simulink model "simulink_RR_adaptive"  (R2024a)
settings: Solver=FixedStepAuto  StartTime=0.0  StopTime=T_max  FixedStep=ST  RelTol=1e-3
values from neighbouring files (symbols this model uses):
  A_m = eye(2)    [init_RR.m]
  alfa = 1    [init_RR.m]
  B_m = eye(2)    [init_RR.m]
  c_11_init = ones(n_q1*n_q2,1)/(n_q1*n_q2)    [init_RR.m]
  c_12_init = ones(n_q1*n_q2,1)/(n_q1*n_q2)    [init_RR.m]
  c_21_init = ones(n_q1*n_q2,1)/(n_q1*n_q2)    [init_RR.m]
  c_22_init = ones(n_q1*n_q2,1)/(n_q1*n_q2)    [init_RR.m]
  delta_q1 = 2*1.1*q_limit/(n_q1-1)    [basis_figure.m]    (also in init_RR.m = 0.345575191895)
  delta_q2 = 2*1.1*q_limit/(n_q2-1)    [basis_figure.m]    (also in init_RR.m = 0.345575191895)
  gamma = 100    [init_RR.m]
  k_m = 1    [init_RR.m]
  k_r = 10    [init_RR.m]
  ksi_m_init = [(l1+l2)/sqrt(2); 0]    [init_RR.m]
  l1 = 4    [init_RR.m]
  l2 = 3    [init_RR.m]
  M = 1000    [init_RR.m]
  mu = 1    [init_RR.m]
  n_q1 = 3    [basis_figure.m]    (also in init_RR.m = 21)
  n_q2 = 3    [basis_figure.m]    (also in init_RR.m = 21)
  omega_r_1 = 5*2*pi/T_ref    (= 0.261799387799)    [init_RR.m]
  omega_r_2 = 7*2*pi/T_ref    (= 0.366519142919)    [init_RR.m]
  q_init = [-pi/4; +pi/4]    [init_RR.m]
  shift1 = ceil(n_q1/2)    [basis_figure.m]    (also in init_RR.m)
  shift2 = ceil(n_q2/2)    [basis_figure.m]    (also in init_RR.m)
  T_max = 300    [init_RR.m]
  u_sat = 5    [init_RR.m]
  VAR_inv = inv(VAR)    [basis_figure.m]    (also in init_RR.m)
settings Model: Creator=gabri  LastModifiedBy=gabri

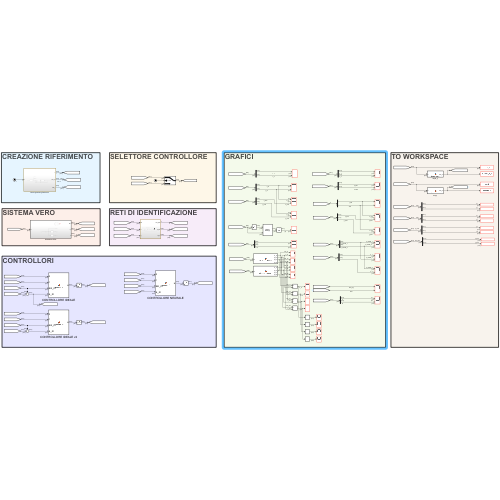
[thumbnail: Simulink's stored preview of the top-level diagram]
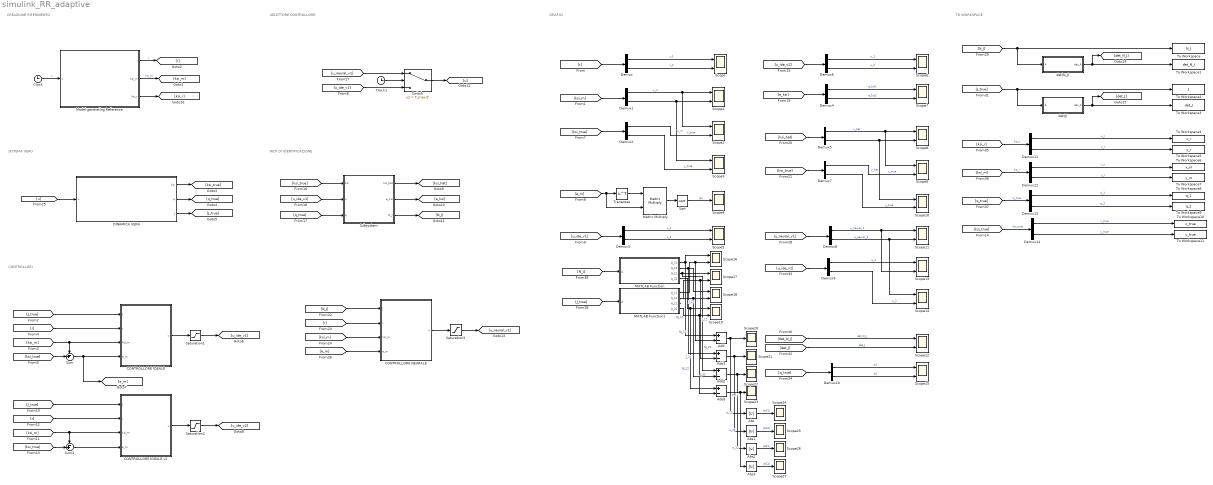
== system simulink_RR_adaptive ==
  note: TO WORKSPACE
  note: CREAZIONE RIFERIMENTO
  note: GRAFICI
  note: SISTEMA VERO
  note: CONTROLLORI
  note: SELETTORE CONTROLLORE
  note: RETI DI IDENTIFICAZIONE
  Abs{,1..3} (4 alike) : Abs  SaturateOnIntegerOverflow=off
  Add{,1..3} (4 alike) : Sum  Inputs=+-
  CONTROLLORE IDEALE : MATLAB Function  TreatAsAtomicUnit=on
  CONTROLLORE IDEALE v2 : MATLAB Function  TreatAsAtomicUnit=on
  CONTROLLORE NEURALE : MATLAB Function  TreatAsAtomicUnit=on
  Clock : Clock
  Clock1 : Clock
  DINAMICA VERA : Subsystem
  Demux{,1..14} (15 alike) : Demux  Outputs=2
  MATLAB Function : MATLAB Function  TreatAsAtomicUnit=on
  MATLAB Function1 : MATLAB Function  TreatAsAtomicUnit=on
  Matrix Multiply : Product  Multiplication=Matrix(*)
  Model generating Reference : Subsystem
  Saturation1 : Saturate  UpperLimit=u_sat  LowerLimit=-u_sat
  Saturation2 : Saturate  UpperLimit=u_sat  LowerLimit=-u_sat
  Saturation3 : Saturate  UpperLimit=u_sat  LowerLimit=-u_sat
  Scope{,1..3,5..19} (19 alike) : Scope  NumInputPorts=2
  Scope{4,20..27} (9 alike) : Scope
  Sqrt : Sqrt
  Subsystem : Subsystem
  Sum : Sum  Inputs=-+|
  Sum1 : Sum  Inputs=-+|
  Switch : Switch  Criteria=u2 > Threshold  Threshold=T_max/2  SaturateOnIntegerOverflow=off  InputSameDT=off
  To Workspace : ToWorkspace  VariableName=N_J  SaveFormat=Timeseries  SampleTime=-1
  To Workspace1 : ToWorkspace  VariableName=det_N_J  SaveFormat=Timeseries  SampleTime=-1
  To Workspace10 : ToWorkspace  VariableName=x_true  SaveFormat=Timeseries  SampleTime=-1
  To Workspace11 : ToWorkspace  VariableName=y_true  SaveFormat=Timeseries  SampleTime=-1
  To Workspace2 : ToWorkspace  VariableName=J  SaveFormat=Timeseries  SampleTime=-1
  To Workspace3 : ToWorkspace  VariableName=det_J  SaveFormat=Timeseries  SampleTime=-1
  To Workspace4 : ToWorkspace  VariableName=x_r  SaveFormat=Timeseries  SampleTime=-1
  To Workspace5 : ToWorkspace  VariableName=y_r  SaveFormat=Timeseries  SampleTime=-1
  To Workspace6 : ToWorkspace  VariableName=x_m  SaveFormat=Timeseries  SampleTime=-1
  To Workspace7 : ToWorkspace  VariableName=y_m  SaveFormat=Timeseries  SampleTime=-1
  To Workspace8 : ToWorkspace  VariableName=q_1  SaveFormat=Timeseries  SampleTime=-1
  To Workspace9 : ToWorkspace  VariableName=q_2  SaveFormat=Timeseries  SampleTime=-1
  Transpose : Math  Operator=transpose
  det(J) : MATLAB Function  TreatAsAtomicUnit=on
  det(N_J) : MATLAB Function  TreatAsAtomicUnit=on
  wires:
  Model generating Reference/2(ksi_m) -> [ksi_m]  "ksi_m"
  Model generating Reference/1(r) -> [r]  "r"
  Clock/1 -> Model generating Reference/1(t)  "t"
  Demux/1 -> Scope/1  "r_1"
  Demux/2 -> Scope/2  "r_2"
  [r] -> Demux/1
  [ksi_m] -> Demux1/1
  Demux1/2 -> Scope3/1, Scope1/2  "y_m"
  Demux1/1 -> Scope2/1, Scope1/1  "x_m"
  [u] -> DINAMICA VERA/1(u)
  DINAMICA VERA/1(ksi) -> [ksi_true]
  DINAMICA VERA/2(q) -> [q_true]
  DINAMICA VERA/3(J) -> [J_true]
  [J_true] -> CONTROLLORE IDEALE/1(J)
  [ksi_m] -> Sum/1, CONTROLLORE IDEALE/3(ksi_m)
  [r] -> CONTROLLORE IDEALE/2(r)
  [ksi_true] -> Sum/2
  Sum/1 -> [e_m], CONTROLLORE IDEALE/4(e_m)
  [u_ide_v1] -> Switch/3
  Switch/1 -> [u]
  [u_neural_v1] -> Switch/1
  [ksi_true] -> Demux2/1
  Demux2/1 -> Scope2/2  "x_true"
  Demux2/2 -> Scope3/2  "y_true"
  [e_m] -> Matrix Multiply/2, Transpose/1
  Transpose/1 -> Matrix Multiply/1
  Matrix Multiply/1 -> Sqrt/1
  Sqrt/1 -> Scope4/1  "|e|"
  [u_ide_v1] -> Demux3/1
  Demux3/1 -> Scope5/1  "u_1"
  Demux3/2 -> Scope5/2  "u_2"
  Sum1/1 -> CONTROLLORE IDEALE v2/4(e_m)
  [ksi_true] -> Sum1/2
  [r] -> CONTROLLORE IDEALE v2/2(r)
  [ksi_m] -> CONTROLLORE IDEALE v2/3(ksi_m), Sum1/1
  [J_true] -> CONTROLLORE IDEALE v2/1(J)
  Demux6/2 -> Scope6/2  "u_2"
  Demux6/1 -> Scope6/1  "u_1"
  [u_ide_v2] -> Demux6/1
  CONTROLLORE IDEALE v2/1(u) -> Saturation2/1
  CONTROLLORE IDEALE/1(u) -> Saturation1/1
  Saturation1/1 -> [u_ide_v1]
  Saturation2/1 -> [u_ide_v2]
  [ksi_true] -> Subsystem/1(ksi)
  [u_ide_v1] -> Subsystem/2(u)
  [q_true] -> Subsystem/3(q)
  Subsystem/1(ksi_hat) -> [ksi_hat]
  Subsystem/2(e_ksi) -> [e_ksi]
  Subsystem/3(N_J) -> [N_J]
  [e_ksi] -> Demux4/1
  Demux4/1 -> Scope7/1  "e_ksi1"
  Demux4/2 -> Scope7/2  "e_ksi2"
  Demux7/2 -> Scope10/2  "y_true"
  Demux7/1 -> Scope9/2  "x_true"
  [ksi_true] -> Demux7/1
  Demux5/1 -> Scope8/1, Scope9/1  "x_hat"
  Demux5/2 -> Scope8/2, Scope10/1  "y_hat"
  [ksi_hat] -> Demux5/1
  Saturation3/1 -> [u_neural_v1]
  CONTROLLORE NEURALE/1(u) -> Saturation3/1
  [N_J] -> CONTROLLORE NEURALE/1(J)
  [r] -> CONTROLLORE NEURALE/2(r)
  [ksi_m] -> CONTROLLORE NEURALE/3(ksi_m)
  [e_m] -> CONTROLLORE NEURALE/4(e_m)
  Clock1/1 -> Switch/2
  Demux8/2 -> Scope11/2, Scope14/1  "u_neural_2"
  Demux8/1 -> Scope13/2, Scope11/1  "u_neural_1"
  [u_neural_v1] -> Demux8/1
  [N_J] -> To Workspace/1, det(N_J)/1(A)
  det(N_J)/1(det_A) -> [det_N_J], To Workspace1/1
  [det_N_J] -> Scope12/1  "det_N_J"
  det(J)/1(det_A) -> To Workspace3/1, [det_J]
  [J_true] -> det(J)/1(A), To Workspace2/1
  [det_J] -> Scope12/2  "det_J"
  Demux9/2 -> Scope14/2  "u_2"
  Demux9/1 -> Scope13/1  "u_1"
  [u_ide_v1] -> Demux9/1
  [q_true] -> Demux10/1
  Demux10/1 -> Scope15/1  "q1"
  Demux10/2 -> Scope15/2  "q2"
  Model generating Reference/3(ksi_r) -> [ksi_r]
  [ksi_r] -> Demux11/1  "ksi_r"
  Demux11/2 -> To Workspace5/1  "y_r"
  Demux11/1 -> To Workspace4/1  "x_r"
  Demux12/1 -> To Workspace6/1  "x_r"
  Demux12/2 -> To Workspace7/1  "y_r"
  [ksi_m] -> Demux12/1  "ksi_r"
  [q_true] -> Demux13/1  "q_true"
  Demux13/1 -> To Workspace8/1  "q_1"
  Demux13/2 -> To Workspace9/1  "q_2"
  Demux14/2 -> To Workspace11/1  "y_true"
  Demux14/1 -> To Workspace10/1  "x_true"
  [ksi_true] -> Demux14/1  "ksi_true"
  [N_J] -> MATLAB Function/1(A)
  [J_true] -> MATLAB Function1/1(A)
  MATLAB Function/1(A_11) -> Add/1, Scope16/1  "NJ_11"
  MATLAB Function/2(A_12) -> Add1/1, Scope17/1  "NJ_12"
  MATLAB Function/3(A_21) -> Add2/1, Scope18/1  "NJ_21"
  MATLAB Function/4(A_22) -> Add3/1, Scope19/1  "NJ_22"
  MATLAB Function1/1(A_11) -> Add/2, Scope16/2  "J_11"
  MATLAB Function1/2(A_12) -> Add1/2, Scope17/2  "J_12"
  MATLAB Function1/3(A_21) -> Add2/2, Scope18/2  "J_21"
  MATLAB Function1/4(A_22) -> Add3/2, Scope19/2  "J_22"
  Add/1 -> Abs/1, Scope20/1  "e_11"
  Add1/1 -> Abs1/1, Scope21/1  "e_12"
  Add2/1 -> Abs2/1, Scope22/1  "e_21"
  Add3/1 -> Abs3/1, Scope23/1  "e_22"
  Abs/1 -> Scope24/1  "|e11|"
  Abs1/1 -> Scope25/1  "|e12|"
  Abs2/1 -> Scope26/1  "|e21|"
  Abs3/1 -> Scope27/1  "|e22|"

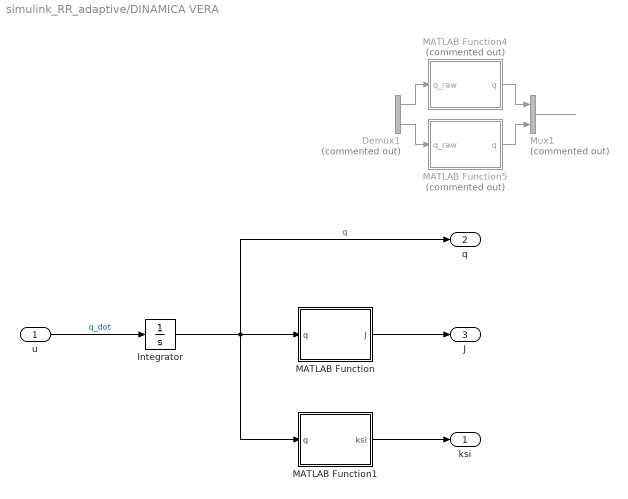
== system simulink_RR_adaptive/DINAMICA VERA ==
  u : Inport
  Demux1 : Demux  Commented=on  Outputs=2
  Integrator : Integrator  InitialCondition=q_init
  MATLAB Function : MATLAB Function  TreatAsAtomicUnit=on
  MATLAB Function1 : MATLAB Function  TreatAsAtomicUnit=on
  MATLAB Function4 : MATLAB Function  Commented=on  TreatAsAtomicUnit=on
  MATLAB Function5 : MATLAB Function  Commented=on  TreatAsAtomicUnit=on
  Mux1 : Mux  Commented=on  Inputs=2
  ksi : Outport
  q : Outport  Port=2
  J : Outport  Port=3
  wires:
  u/1 -> Integrator/1  "q_dot"
  Integrator/1 -> q/1, MATLAB Function1/1(q), MATLAB Function/1(q)  "q"
  MATLAB Function1/1(ksi) -> ksi/1
  MATLAB Function/1(J) -> J/1
  Demux1/2 -> MATLAB Function5/1(q_raw)
  Demux1/1 -> MATLAB Function4/1(q_raw)
  MATLAB Function5/1(q) -> Mux1/2
  MATLAB Function4/1(q) -> Mux1/1
  Mux1/1 -> ?

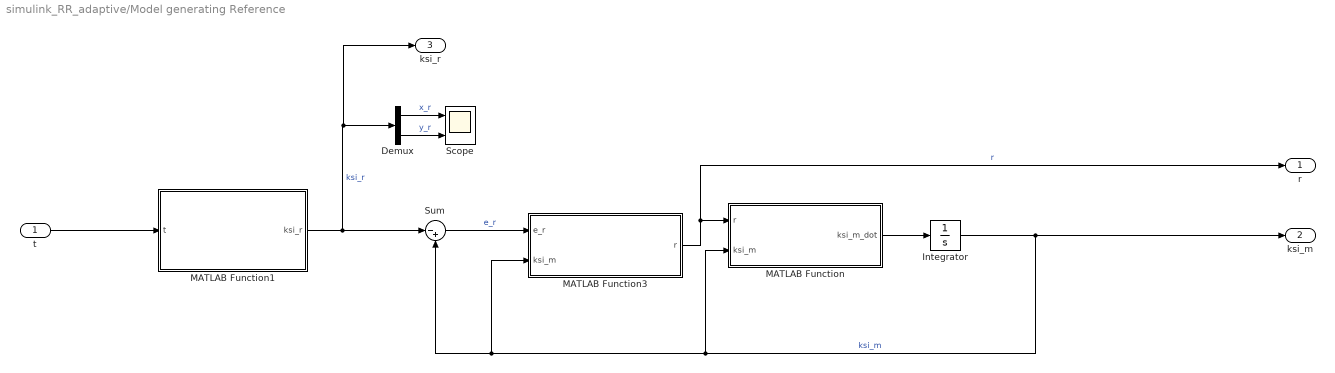
== system simulink_RR_adaptive/Model generating Reference ==
  t : Inport
  Demux : Demux  Outputs=2
  Integrator : Integrator  InitialCondition=ksi_m_init
  MATLAB Function : MATLAB Function  TreatAsAtomicUnit=on
  MATLAB Function1 : MATLAB Function  TreatAsAtomicUnit=on
  MATLAB Function3 : MATLAB Function  TreatAsAtomicUnit=on
  Scope : Scope  NumInputPorts=2
  Sum : Sum  Inputs=|-+
  r : Outport
  ksi_m : Outport  Port=2
  ksi_r : Outport  Port=3
  wires:
  MATLAB Function1/1(ksi_r) -> ksi_r/1, Demux/1, Sum/1  "ksi_r"
  Integrator/1 -> ksi_m/1, MATLAB Function3/2(ksi_m), Sum/2, MATLAB Function/2(ksi_m)  "ksi_m"
  t/1 -> MATLAB Function1/1(t)
  MATLAB Function3/1(r) -> r/1, MATLAB Function/1(r)  "r"
  MATLAB Function/1(ksi_m_dot) -> Integrator/1
  Sum/1 -> MATLAB Function3/1(e_r)  "e_r"
  Demux/1 -> Scope/1  "x_r"
  Demux/2 -> Scope/2  "y_r"

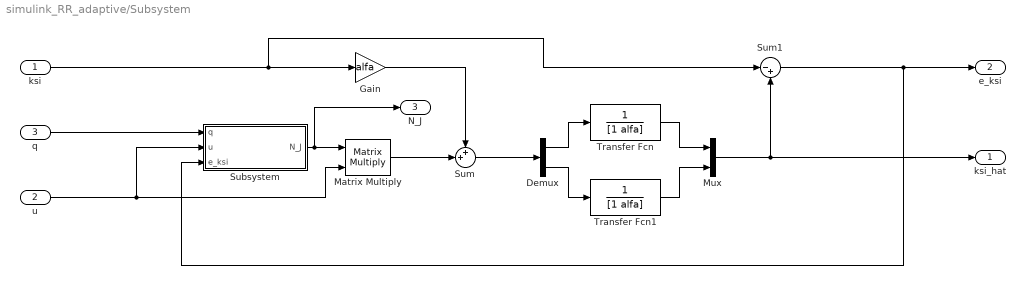
== system simulink_RR_adaptive/Subsystem ==
  ksi : Inport
  u : Inport  Port=2
  q : Inport  Port=3
  Demux : Demux  Outputs=2
  Gain : Gain  Gain=alfa
  Matrix Multiply : Product  Multiplication=Matrix(*)
  Mux : Mux  Inputs=2
  Subsystem : Subsystem
  Sum : Sum  Inputs=++|
  Sum1 : Sum  Inputs=|-+
  Transfer Fcn : TransferFcn  Denominator=[1 alfa]
  Transfer Fcn1 : TransferFcn  Denominator=[1 alfa]
  ksi_hat : Outport
  e_ksi : Outport  Port=2
  N_J : Outport  Port=3
  wires:
  ksi/1 -> Sum1/1, Gain/1
  q/1 -> Subsystem/1(q)
  u/1 -> Matrix Multiply/2, Subsystem/2(u)
  Subsystem/1(N_J) -> N_J/1, Matrix Multiply/1
  Matrix Multiply/1 -> Sum/2
  Gain/1 -> Sum/1
  Sum/1 -> Demux/1
  Demux/1 -> Transfer Fcn/1
  Demux/2 -> Transfer Fcn1/1
  Transfer Fcn/1 -> Mux/1
  Transfer Fcn1/1 -> Mux/2
  Mux/1 -> ksi_hat/1, Sum1/2
  Sum1/1 -> Subsystem/3(e_ksi), e_ksi/1

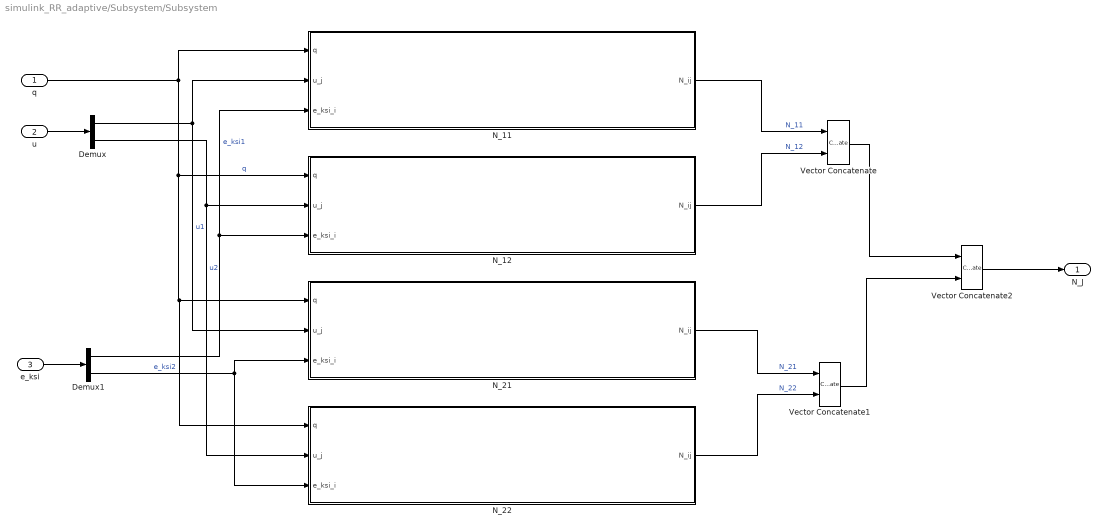
== system simulink_RR_adaptive/Subsystem/Subsystem ==
  q : Inport
  u : Inport  Port=2
  e_ksi : Inport  Port=3
  Demux : Demux  Outputs=2
  Demux1 : Demux  Outputs=2
  N_11 : Subsystem
  N_12 : Subsystem
  N_21 : Subsystem
  N_22 : Subsystem
  Vector Concatenate : Concatenate  Mode=Multidimensional array  ConcatenateDimension=2
  Vector Concatenate1 : Concatenate  Mode=Multidimensional array  ConcatenateDimension=2
  Vector Concatenate2 : Concatenate  Mode=Multidimensional array
  N_J : Outport
  wires:
  u/1 -> Demux/1
  Demux/1 -> N_21/2(u_j), N_11/2(u_j)  "u1"
  Demux/2 -> N_22/2(u_j), N_12/2(u_j)  "u2"
  e_ksi/1 -> Demux1/1
  Demux1/1 -> N_12/3(e_ksi_i), N_11/3(e_ksi_i)  "e_ksi1"
  Demux1/2 -> N_22/3(e_ksi_i), N_21/3(e_ksi_i)  "e_ksi2"
  q/1 -> N_22/1(q), N_21/1(q), N_12/1(q), N_11/1(q)  "q"
  N_12/1(N_ij) -> Vector Concatenate/2  "N_12"
  N_21/1(N_ij) -> Vector Concatenate1/1  "N_21"
  Vector Concatenate/1 -> Vector Concatenate2/1
  Vector Concatenate1/1 -> Vector Concatenate2/2
  Vector Concatenate2/1 -> N_J/1
  N_22/1(N_ij) -> Vector Concatenate1/2  "N_22"
  N_11/1(N_ij) -> Vector Concatenate/1  "N_11"

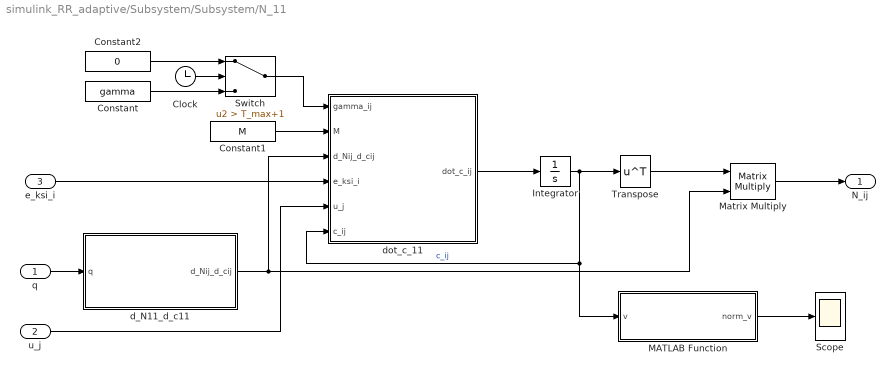
== system simulink_RR_adaptive/Subsystem/Subsystem/N_11 ==
  q : Inport
  u_j : Inport  Port=2
  e_ksi_i : Inport  Port=3
  Clock : Clock
  Constant : Constant  Value=gamma
  Constant1 : Constant  Value=M
  Constant2 : Constant  Value=0
  Integrator : Integrator  InitialCondition=c_11_init
  MATLAB Function : MATLAB Function  TreatAsAtomicUnit=on
  Matrix Multiply : Product  Multiplication=Matrix(*)
  Scope : Scope
  Switch : Switch  Criteria=u2 > Threshold  Threshold=T_max+1  SaturateOnIntegerOverflow=off  InputSameDT=off
  Transpose : Math  Operator=transpose
  d_N11_d_c11 : MATLAB Function  TreatAsAtomicUnit=on
  dot_c_11 : MATLAB Function  TreatAsAtomicUnit=on
  N_ij : Outport
  wires:
  Matrix Multiply/1 -> N_ij/1
  q/1 -> d_N11_d_c11/1(q)
  d_N11_d_c11/1(d_Nij_d_cij) -> Matrix Multiply/2, dot_c_11/3(d_Nij_d_cij)
  Transpose/1 -> Matrix Multiply/1
  Integrator/1 -> MATLAB Function/1(v), dot_c_11/6(c_ij), Transpose/1  "c_ij"
  dot_c_11/1(dot_c_ij) -> Integrator/1
  u_j/1 -> dot_c_11/5(u_j)
  e_ksi_i/1 -> dot_c_11/4(e_ksi_i)
  Constant1/1 -> dot_c_11/2(M)
  MATLAB Function/1(norm_v) -> Scope/1
  Constant/1 -> Switch/3
  Constant2/1 -> Switch/1
  Clock/1 -> Switch/2
  Switch/1 -> dot_c_11/1(gamma_ij)

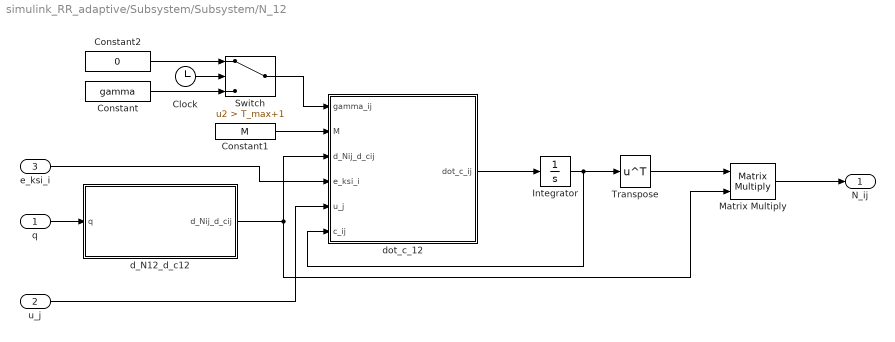
== system simulink_RR_adaptive/Subsystem/Subsystem/N_12 ==
  q : Inport
  u_j : Inport  Port=2
  e_ksi_i : Inport  Port=3
  Clock : Clock
  Constant : Constant  Value=gamma
  Constant1 : Constant  Value=M
  Constant2 : Constant  Value=0
  Integrator : Integrator  InitialCondition=c_12_init
  Matrix Multiply : Product  Multiplication=Matrix(*)
  Switch : Switch  Criteria=u2 > Threshold  Threshold=T_max+1  SaturateOnIntegerOverflow=off  InputSameDT=off
  Transpose : Math  Operator=transpose
  d_N12_d_c12 : MATLAB Function  TreatAsAtomicUnit=on
  dot_c_12 : MATLAB Function  TreatAsAtomicUnit=on
  N_ij : Outport
  wires:
  e_ksi_i/1 -> dot_c_12/4(e_ksi_i)
  u_j/1 -> dot_c_12/5(u_j)
  dot_c_12/1(dot_c_ij) -> Integrator/1
  Integrator/1 -> dot_c_12/6(c_ij), Transpose/1
  Transpose/1 -> Matrix Multiply/1
  d_N12_d_c12/1(d_Nij_d_cij) -> dot_c_12/3(d_Nij_d_cij), Matrix Multiply/2
  q/1 -> d_N12_d_c12/1(q)
  Matrix Multiply/1 -> N_ij/1
  Constant1/1 -> dot_c_12/2(M)
  Constant2/1 -> Switch/1
  Constant/1 -> Switch/3
  Clock/1 -> Switch/2
  Switch/1 -> dot_c_12/1(gamma_ij)

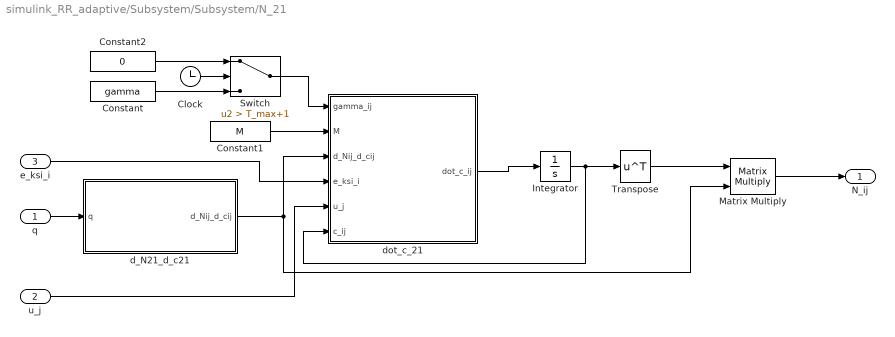
== system simulink_RR_adaptive/Subsystem/Subsystem/N_21 ==
  q : Inport
  u_j : Inport  Port=2
  e_ksi_i : Inport  Port=3
  Clock : Clock
  Constant : Constant  Value=gamma
  Constant1 : Constant  Value=M
  Constant2 : Constant  Value=0
  Integrator : Integrator  InitialCondition=c_21_init
  Matrix Multiply : Product  Multiplication=Matrix(*)
  Switch : Switch  Criteria=u2 > Threshold  Threshold=T_max+1  SaturateOnIntegerOverflow=off  InputSameDT=off
  Transpose : Math  Operator=transpose
  d_N21_d_c21 : MATLAB Function  TreatAsAtomicUnit=on
  dot_c_21 : MATLAB Function  TreatAsAtomicUnit=on
  N_ij : Outport
  wires:
  Matrix Multiply/1 -> N_ij/1
  q/1 -> d_N21_d_c21/1(q)
  d_N21_d_c21/1(d_Nij_d_cij) -> Matrix Multiply/2, dot_c_21/3(d_Nij_d_cij)
  Transpose/1 -> Matrix Multiply/1
  Integrator/1 -> dot_c_21/6(c_ij), Transpose/1
  dot_c_21/1(dot_c_ij) -> Integrator/1
  u_j/1 -> dot_c_21/5(u_j)
  e_ksi_i/1 -> dot_c_21/4(e_ksi_i)
  Constant1/1 -> dot_c_21/2(M)
  Constant2/1 -> Switch/1
  Constant/1 -> Switch/3
  Clock/1 -> Switch/2
  Switch/1 -> dot_c_21/1(gamma_ij)

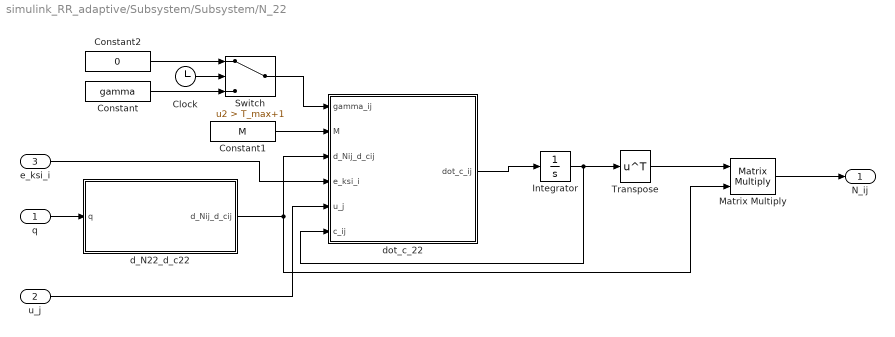
== system simulink_RR_adaptive/Subsystem/Subsystem/N_22 ==
  q : Inport
  u_j : Inport  Port=2
  e_ksi_i : Inport  Port=3
  Clock : Clock
  Constant : Constant  Value=gamma
  Constant1 : Constant  Value=M
  Constant2 : Constant  Value=0
  Integrator : Integrator  InitialCondition=c_22_init
  Matrix Multiply : Product  Multiplication=Matrix(*)
  Switch : Switch  Criteria=u2 > Threshold  Threshold=T_max+1  SaturateOnIntegerOverflow=off  InputSameDT=off
  Transpose : Math  Operator=transpose
  d_N22_d_c22 : MATLAB Function  TreatAsAtomicUnit=on
  dot_c_22 : MATLAB Function  TreatAsAtomicUnit=on
  N_ij : Outport
  wires:
  e_ksi_i/1 -> dot_c_22/4(e_ksi_i)
  u_j/1 -> dot_c_22/5(u_j)
  dot_c_22/1(dot_c_ij) -> Integrator/1
  Integrator/1 -> dot_c_22/6(c_ij), Transpose/1
  Transpose/1 -> Matrix Multiply/1
  d_N22_d_c22/1(d_Nij_d_cij) -> dot_c_22/3(d_Nij_d_cij), Matrix Multiply/2
  q/1 -> d_N22_d_c22/1(q)
  Matrix Multiply/1 -> N_ij/1
  Constant1/1 -> dot_c_22/2(M)
  Constant2/1 -> Switch/1
  Constant/1 -> Switch/3
  Clock/1 -> Switch/2
  Switch/1 -> dot_c_22/1(gamma_ij)

== matlab function simulink_RR_adaptive/Model generating Reference/MATLAB Function1 ==
  data: t input; ksi_r output; l1 parameter; l2 parameter; omega_r_1 parameter; omega_r_2 parameter
function ksi_r  = ksi_ref(t, l1, l2, omega_r_1, omega_r_2)

x_r = (1/sqrt(2))*(l1+l2)*cos(omega_r_1*t);

y_r = 0.5*(1/sqrt(2))*(l1+l2)*(1 + 0.5*sin(omega_r_2*t));

ksi_r = [x_r; y_r];

== matlab function simulink_RR_adaptive/Subsystem/Subsystem/N_12/dot_c_12 ==
  data: gamma_ij input; M input; dot_c_ij output; d_Nij_d_cij input; e_ksi_i input; u_j input; c_ij input
function dot_c_ij = dot_c_ij(gamma_ij, M, d_Nij_d_cij, e_ksi_i, u_j, c_ij)

if norm(c_ij) <= M
    dot_c_ij = - gamma_ij * d_Nij_d_cij * e_ksi_i * u_j;
else
    dot_c_ij = - gamma_ij * d_Nij_d_cij * e_ksi_i * u_j + gamma_ij * c_ij' * d_Nij_d_cij * e_ksi_i * u_j * (1/norm(c_ij)^2) * c_ij;
end

== matlab function simulink_RR_adaptive/Model generating Reference/MATLAB Function ==
  data: r input; ksi_m_dot output; ksi_m input; B_m parameter; A_m parameter
function ksi_m_dot = reference_dynamic(r, ksi_m, B_m, A_m)

ksi_m_dot = -A_m*ksi_m + B_m*r;

== matlab function simulink_RR_adaptive/Model generating Reference/MATLAB Function3 ==
  data: e_r input; r output; ksi_m input; k_r parameter; B_m parameter; A_m parameter
function r = reference_controller(e_r, ksi_m, k_r, B_m, A_m)

r = B_m\(A_m*ksi_m - k_r*e_r);

== matlab function simulink_RR_adaptive/CONTROLLORE IDEALE ==
  data: J input; r input; ksi_m input; u output; e_m input; k_m parameter; B_m parameter; A_m parameter
function u = controllore_V1(J, r, ksi_m, e_m, k_m, B_m, A_m)

u = J\(-A_m*ksi_m + B_m*r - k_m*e_m);

== matlab function simulink_RR_adaptive/DINAMICA VERA/MATLAB Function1 ==
  data: q input; ksi output; l2 parameter; l1 parameter
function ksi = Q(q, l2, l1)

q1 = q(1);
q2 = q(2);

x = l1*cos(q1) + l2*cos(q1 + q2);
y = l1*sin(q1) + l2*sin(q1 + q2);

ksi = [x; y];

== matlab function simulink_RR_adaptive/Subsystem/Subsystem/N_21/d_N21_d_c21 ==
  data: q input; d_Nij_d_cij output; VAR_inv parameter; delta_q2 parameter; delta_q1 parameter; shift2 parameter; shift1 parameter; n_q2 parameter; n_q1 parameter
function d_Nij_d_cij = d_Nij_d_cij(q, VAR_inv, delta_q2, delta_q1, shift2, shift1, n_q2, n_q1)

d_Nij_d_cij = zeros(n_q1*n_q2, 1);

for i = 1:length(d_Nij_d_cij)

    k = ceil(i/n_q1);
    p = mod(i+n_q1-1, n_q1)+1;

    centro_kp = [(k - shift1)*delta_q1; (p - shift2)*delta_q2];

    d_Nij_d_cij(i) = exp(-0.5*(q - centro_kp)'*VAR_inv*(q - centro_kp));

end

== matlab function simulink_RR_adaptive/Subsystem/Subsystem/N_21/dot_c_21 ==
  data: gamma_ij input; M input; dot_c_ij output; d_Nij_d_cij input; e_ksi_i input; u_j input; c_ij input
function dot_c_ij = dot_c_ij(gamma_ij, M, d_Nij_d_cij, e_ksi_i, u_j, c_ij)

if norm(c_ij) <= M
    dot_c_ij = - gamma_ij * d_Nij_d_cij * e_ksi_i * u_j;
else
    dot_c_ij = - gamma_ij * d_Nij_d_cij * e_ksi_i * u_j + gamma_ij * c_ij' * d_Nij_d_cij * e_ksi_i * u_j * (1/norm(c_ij)^2) * c_ij;
end

== matlab function simulink_RR_adaptive/Subsystem/Subsystem/N_22/d_N22_d_c22 ==
  data: q input; d_Nij_d_cij output; VAR_inv parameter; delta_q2 parameter; delta_q1 parameter; shift2 parameter; shift1 parameter; n_q2 parameter; n_q1 parameter
function d_Nij_d_cij = d_Nij_d_cij(q, VAR_inv, delta_q2, delta_q1, shift2, shift1, n_q2, n_q1)

d_Nij_d_cij = zeros(n_q1*n_q2, 1);

for i = 1:length(d_Nij_d_cij)

    k = ceil(i/n_q1);
    p = mod(i+n_q1-1, n_q1)+1;

    centro_kp = [(k - shift1)*delta_q1; (p - shift2)*delta_q2];

    d_Nij_d_cij(i) = exp(-0.5*(q - centro_kp)'*VAR_inv*(q - centro_kp));

end

== matlab function simulink_RR_adaptive/Subsystem/Subsystem/N_22/dot_c_22 ==
  data: gamma_ij input; M input; dot_c_ij output; d_Nij_d_cij input; e_ksi_i input; u_j input; c_ij input
function dot_c_ij = dot_c_ij(gamma_ij, M, d_Nij_d_cij, e_ksi_i, u_j, c_ij)

if norm(c_ij) <= M
    dot_c_ij = - gamma_ij * d_Nij_d_cij * e_ksi_i * u_j;
else
    dot_c_ij = - gamma_ij * d_Nij_d_cij * e_ksi_i * u_j + gamma_ij * c_ij' * d_Nij_d_cij * e_ksi_i * u_j * (1/norm(c_ij)^2) * c_ij;
end

== matlab function simulink_RR_adaptive/CONTROLLORE NEURALE ==
  data: J input; r input; ksi_m input; u output; e_m input; k_m parameter; B_m parameter; A_m parameter
function u = controllore_V1(J, r, ksi_m, e_m, k_m, B_m, A_m)

u = J\(-A_m*ksi_m + B_m*r - k_m*e_m);

== matlab function simulink_RR_adaptive/det(N_J) ==
  data: A input; det_A output
function det_A = determinant(A)

det_A = det(A);

== matlab function simulink_RR_adaptive/det(J) ==
  data: A input; det_A output
function det_A = determinant(A)

det_A = det(A);

== matlab function simulink_RR_adaptive/Subsystem/Subsystem/N_11/MATLAB Function ==
  data: v input; norm_v output
function norm_v = norm(v)

norm_v = norm(v);

== matlab function simulink_RR_adaptive/DINAMICA VERA/MATLAB Function ==
  data: q input; J output; l1 parameter; l2 parameter
function J = jacobiano(q, l1, l2)

q1 = q(1);
q2 = q(2);

J = [-l1*sin(q1) - l2*sin(q1 + q2),   -l2*sin(q1 + q2);
      l1*cos(q1) + l2*cos(q1 + q2),    l2*cos(q1 + q2)];

== matlab function simulink_RR_adaptive/MATLAB Function ==
  data: A input; A_11 output; A_12 output; A_21 output; A_22 output
function [A_11, A_12, A_21, A_22] = element_extractor(A)

A_11 = A(1,1);
A_12 = A(1,2);
A_21 = A(2,1);
A_22 = A(2,2);

== matlab function simulink_RR_adaptive/MATLAB Function1 ==
  data: A input; A_11 output; A_12 output; A_21 output; A_22 output
function [A_11, A_12, A_21, A_22] = element_extractor(A)

A_11 = A(1,1);
A_12 = A(1,2);
A_21 = A(2,1);
A_22 = A(2,2);

== matlab function simulink_RR_adaptive/CONTROLLORE IDEALE v2 ==
  data: J input; r input; ksi_m input; u output; e_m input; k_m parameter; B_m parameter; A_m parameter; mu parameter
function u = controllore_V2(J, r, ksi_m, e_m, k_m, B_m, A_m, mu)

u = J'*(J*J' + mu*eye(2))\(-A_m*ksi_m + B_m*r - k_m*e_m);

== matlab function simulink_RR_adaptive/Subsystem/Subsystem/N_11/dot_c_11 ==
  data: gamma_ij input; M input; dot_c_ij output; d_Nij_d_cij input; e_ksi_i input; u_j input; c_ij input
function dot_c_ij = dot_c_ij(gamma_ij, M, d_Nij_d_cij, e_ksi_i, u_j, c_ij)

if norm(c_ij) <= M
    dot_c_ij = - gamma_ij * d_Nij_d_cij * e_ksi_i * u_j;
else
    dot_c_ij = - gamma_ij * d_Nij_d_cij * e_ksi_i * u_j + gamma_ij * c_ij' * d_Nij_d_cij * e_ksi_i * u_j * (1/norm(c_ij)^2) * c_ij;
end

== matlab function simulink_RR_adaptive/DINAMICA VERA/MATLAB Function4 ==
  data: q_raw input; q output
function q = wrap_to_pi(q_raw)

q = atan2(sin(q_raw), cos(q_raw));

== matlab function simulink_RR_adaptive/DINAMICA VERA/MATLAB Function5 ==
  data: q_raw input; q output
function q = wrap_to_pi(q_raw)

q = atan2(sin(q_raw), cos(q_raw));

== matlab function simulink_RR_adaptive/Subsystem/Subsystem/N_11/d_N11_d_c11 ==
  data: q input; d_Nij_d_cij output; VAR_inv parameter; delta_q2 parameter; delta_q1 parameter; shift2 parameter; shift1 parameter; n_q2 parameter; n_q1 parameter
function d_Nij_d_cij = d_Nij_d_cij(q, VAR_inv, delta_q2, delta_q1, shift2, shift1, n_q2, n_q1)

d_Nij_d_cij = zeros(n_q1*n_q2, 1);

for i = 1:length(d_Nij_d_cij)

    k = ceil(i/n_q1);
    p = mod(i+n_q1-1, n_q1)+1;

    centro_kp = [(k - shift1)*delta_q1; (p - shift2)*delta_q2];

    d_Nij_d_cij(i) = exp(-0.5*(q - centro_kp)'*VAR_inv*(q - centro_kp));

end

== matlab function simulink_RR_adaptive/Subsystem/Subsystem/N_12/d_N12_d_c12 ==
  data: q input; d_Nij_d_cij output; VAR_inv parameter; delta_q2 parameter; delta_q1 parameter; shift2 parameter; shift1 parameter; n_q2 parameter; n_q1 parameter
function d_Nij_d_cij = d_Nij_d_cij(q, VAR_inv, delta_q2, delta_q1, shift2, shift1, n_q2, n_q1)

d_Nij_d_cij = zeros(n_q1*n_q2, 1);

for i = 1:length(d_Nij_d_cij)

    k = ceil(i/n_q1);
    p = mod(i+n_q1-1, n_q1)+1;

    centro_kp = [(k - shift1)*delta_q1; (p - shift2)*delta_q2];

    d_Nij_d_cij(i) = exp(-0.5*(q - centro_kp)'*VAR_inv*(q - centro_kp));

end
